simulink model "NER_Cold_Hub_A13_PCM"  (R2025a)
settings: Solver=VariableStepAuto  StartTime=0.0  StopTime=64800  RelTol=1e-3
settings Model: Creator=Victus  LastModifiedBy=Victus

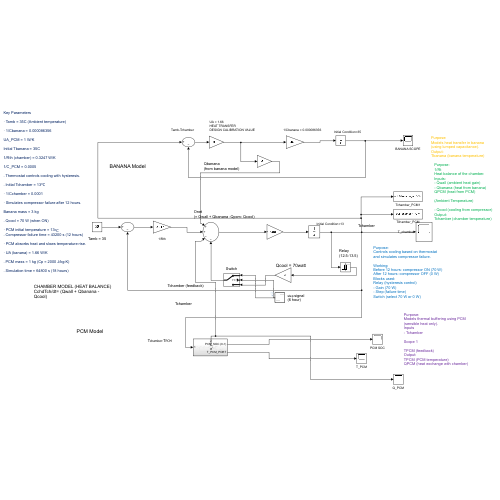
[thumbnail: Simulink's stored preview of the top-level diagram]
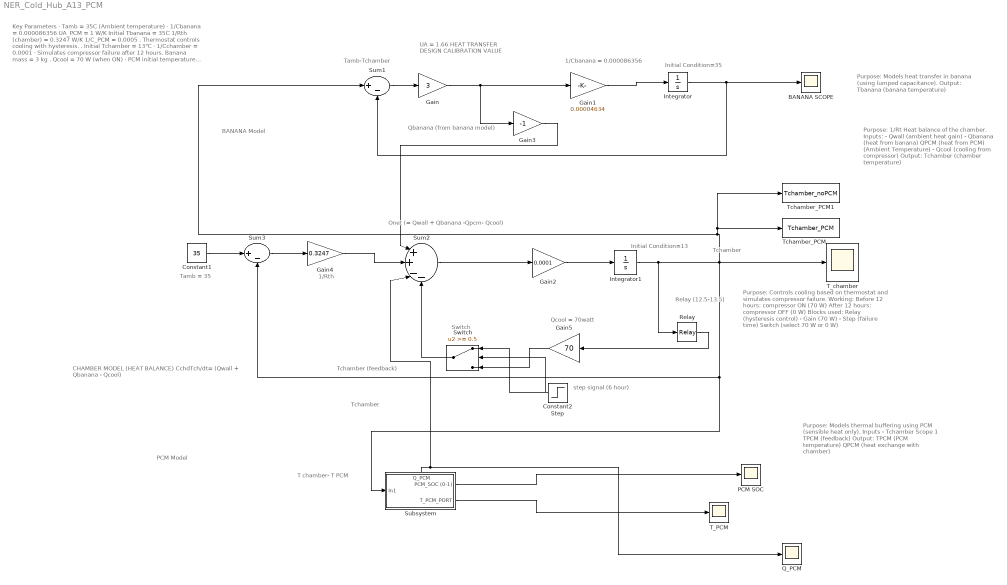
== system NER_Cold_Hub_A13_PCM ==
  note: Purpose:
      | 1/Rt
      | Heat balance of the chamber.
      | Inputs:
      | - Qwall (ambient heat gain)
      | - Qbanana (heat from banana)
      | QPCM (heat from PCM)
      |
      | (Ambient Temperature)
      |
      | - Qcool (cooling from compressor)
      | Output:
      | Tchamber (chamber temperature)
  note: BANANA Model
  note: 1/Rth
  note: UA = 1.66
      | HEAT TRANSFER
      | DESIGN CALIBRATION VALUE
  note: Initial Condition=13
  note: Qcool = 70watt
  note: 1/Cbanana = 0.000086356
  note: Tchamber
  note: Qbanana
      | (from banana model)
  note: Tamb = 35
  note: Tamb-Tchamber
  note: Onet
      | (= Qwall + Qbanana -Qpcm- Qcool)
  note: Switch
  note: Relay
      | (12.5-13.5)
  note: Purpose:
      | Controls cooling based on thermostat
      | and simulates compressor failure.
      |
      | Working:
      | Before 12 hours: compressor ON (70 W)
      | After 12 hours: compressor OFF (0 W)
      | Blocks used:
      | Relay (hysteresis control)
      | - Gain (70 W)
      | - Step (failure time)
      | Switch (select 70 W or 0 W)
  note: step signal
      | (6 hour)
  note: Initial Condition=35
  note: Tchamber
  note: Key Parameters
      |
      | · Tamb = 35C (Ambient temperature)
      |
      | · 1/Cbanana = 0.000086356
      |
      | UA_PCM = 1 W/K
      |
      | Initial Tbanana = 35C
      |
      | 1/Rth (chamber) = 0.3247 W/K
      |
      | 1/C_PCM = 0.0005
      |
      | . Thermostat controls cooling with hysteresis.
      |
      | . Initial Tchamber = 13℃
      |
      | · 1/Cchamber = 0.0001
      |
      | · Simulates compressor failure after 12 hours.
      |
      | Banana mass = 3 kg
      |
      | . Qcool = 70 W (when ON)
      |
      | · PCM initial temperature = 13℃
      | . Compressor failure time = 43200 s (12 hours)
      |
      | · PCM absorbs heat and slows temperature rise.
      |
      | · UA (banana) = 1.66 W/K
      |
      | . PCM mass = 1 kg (Cp = 2000 J/kg-K)
      |
      | . Simulation time = 64800 s (18 hours)
  note: CHAMBER MODEL (HEAT BALANCE)
      | CchdTch/dt= (Qwall + Qbanana - Qcool)
  note: PCM Model
  note: Purpose:
      | Models heat transfer in banana
      | (using lumped capacitance).
      | Output:
      | Tbanana (banana temperature)
  note: Tchamber (feedback)
  note: T chamber- T PCM
  note: Purpose:
      | Models thermal buffering using PCM
      | (sensible heat only).
      | Inputs
      | - Tchamber
      |
      | Scope 1
      |
      | TPCM (feedback)
      | Output:
      | TPCM (PCM temperature)
      | QPCM (heat exchange with chamber)
  BANANA SCOPE : Scope
      settings: ActiveDisplayYMinimum=10.334852167377413  ActiveDisplayYMaximum=37.74057198140251
  Constant1 : Constant  Value=35
  Constant2 : Constant  Value=0
  Gain : Gain  Gain=3
  Gain1 : Gain  Gain=0.00004634
  Gain2 : Gain  Gain=0.0001
  Gain3 : Gain  Gain=-1
  Gain4 : Gain  Gain=0.3247
  Gain5 : Gain  Gain=70
  Integrator : Integrator  InitialCondition=35
  Integrator1 : Integrator  InitialCondition=13
  PCM SOC : Scope
      settings: ActiveDisplayYMinimum=0.48325003857793658  ActiveDisplayYMaximum=1.0574166623802292  DataLoggingVariableName=ScopeData3
  Q_PCM : Scope
      settings: ActiveDisplayYMinimum=-2.3897501458159094  ActiveDisplayYMaximum=6.5077513123277315  DataLoggingVariableName=ScopeData2
  Relay : Relay  OnSwitchValue=13.5  OffSwitchValue=12.5
  Step : Step  Time=43200  SampleTime=0
  Subsystem : Subsystem
      settings: PortSchema="{\"entries\":[{\"content\":{\"sides\":[{\"content\":{\"connectorIds\":[\"In1\"]},\"type\":\"ConnectorPlacement.EquallySpacedRectSide\",\"uuid\":\"4ee914d6-cfaa-4935-95bf-23db2b0812a2\"},{\"content\":{\"connectorIds\":[\"Out1\",\"Out2\"],\"side\":\"RIGHT\"},\"type\":\"ConnectorPlacement.EquallySpacedRectSide\",\"uuid\":\"3445636c-8e97-40dc-8415-16fea3a7e5a4\"},{\"content\":{\"connectorIds\":[\"Out3\"],\"side\":\"TOP\"},\"type\":\"ConnectorPlacement.EquallySpacedRectSide\",\"uuid\":\"adb7bce1-8bd6-4c94-ab0d-bbc94c03674c\"}]},\"type\":\"ConnectorPlacement.EquallySpacedConnector\",\"uuid\":\"4763e0d7-e2fa-4df5-8b70-4a2f3a1c411a\"}],\"packageUris\":[\"http://schema.mathworks.com/mf0/Connector/R2020b\"],\"version\":\"1.0\"}"
  Sum1 : Sum  Inputs=|+-
  Sum2 : Sum  Inputs=|++--
  Sum3 : Sum  Inputs=|+-
  Switch : Switch  Threshold=0.5  SaturateOnIntegerOverflow=off  InputSameDT=off
  T_PCM : Scope
      settings: ActiveDisplayYMinimum=3  ActiveDisplayYMaximum=23  DataLoggingVariableName=ScopeData4
  T_chamber : Scope
      settings: ActiveDisplayYMinimum=10.203013239330566  ActiveDisplayYMaximum=33.172880845998385
  Tchamber_PCM : ToWorkspace  VariableName=Tchamber_PCM  SaveFormat=Timeseries  SampleTime=-1
  Tchamber_PCM1 : ToWorkspace  VariableName=Tchamber_noPCM  SaveFormat=Timeseries  SampleTime=-1
  wires:
  Sum1/1 -> Gain/1
  Gain/1 -> Gain3/1, Gain1/1
  Integrator/1 -> Sum1/2, BANANA SCOPE/1
  Gain3/1 -> Sum2/1
  Integrator1/1 -> Subsystem/1(In1), Sum3/2, T_chamber/1, Tchamber_PCM1/1, Tchamber_PCM/1, Sum1/1, Relay/1
  Step/1 -> Switch/2
  Constant2/1 -> Switch/1
  Gain4/1 -> Sum2/2
  Switch/1 -> Sum2/4
  Sum3/1 -> Gain4/1
  Gain2/1 -> Integrator1/1
  Gain1/1 -> Integrator/1
  Gain5/1 -> Switch/3
  Sum2/1 -> Gain2/1
  Relay/1 -> Gain5/1
  Constant1/1 -> Sum3/1
  Subsystem/3(Q_PCM) -> Q_PCM/1, Sum2/3
  Subsystem/1(PCM_SOC (0-1)) -> PCM SOC/1
  Subsystem/2(T_PCM_PORT) -> T_PCM/1

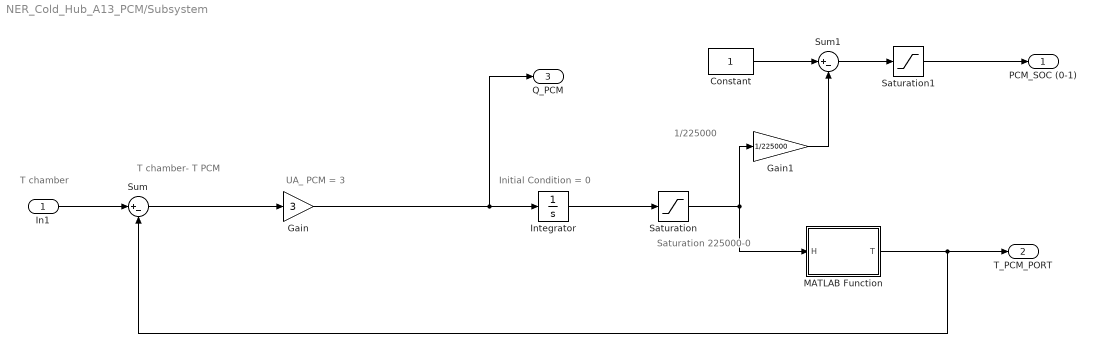
== system NER_Cold_Hub_A13_PCM/Subsystem ==
  note: 1/225000
  note: Saturation
      | 225000-0
  note: Initial Condition = 0
  note: UA_ PCM = 3
  note: T chamber- T PCM
  note: T chamber
  In1 : Inport
  Constant : Constant
  Gain : Gain  Gain=3
  Gain1 : Gain  Gain=1/225000
  Integrator : Integrator
  MATLAB Function : MATLAB Function  TreatAsAtomicUnit=on
  Saturation : Saturate  UpperLimit=1e9  LowerLimit=0
  Saturation1 : Saturate  UpperLimit=1  LowerLimit=0
  Sum : Sum  Inputs=|+-
  Sum1 : Sum  Inputs=|+-
  PCM_SOC (0-1) : Outport
  T_PCM_PORT : Outport  Port=2
  Q_PCM : Outport  Port=3
  wires:
  Sum/1 -> Gain/1
  Integrator/1 -> Saturation/1
  Gain/1 -> Q_PCM/1, Integrator/1
  Saturation/1 -> Gain1/1, MATLAB Function/1(H)
  MATLAB Function/1(T) -> Sum/2, T_PCM_PORT/1
  Sum1/1 -> Saturation1/1
  Constant/1 -> Sum1/1
  Gain1/1 -> Sum1/2
  Saturation1/1 -> PCM_SOC (0-1)/1
  In1/1 -> Sum/1

== matlab function NER_Cold_Hub_A13_PCM/Subsystem/MATLAB Function ==
  data: H input; T output
function T = pcm_temperature(H)

m = 1;
L = 225000;
Cp_s = 2160;
Cp_l = 2160;
T_m = 13;

H_max = m*L;

if H <= 0
    T = T_m;

elseif H < H_max
    T = T_m;

else
    T = T_m + (H-H_max)/(m*Cp_l);
end
